simulink model "Car"  (R2022b)
settings: Solver=VariableStepAuto  StartTime=0.0  StopTime=10.0  RelTol=1e-3
libraries: slpidlib x1
settings Model: Creator=Shayan  LastModifiedBy=Shayan
settings DebuggingCC: UnderSpecifiedDimensionMsg=error

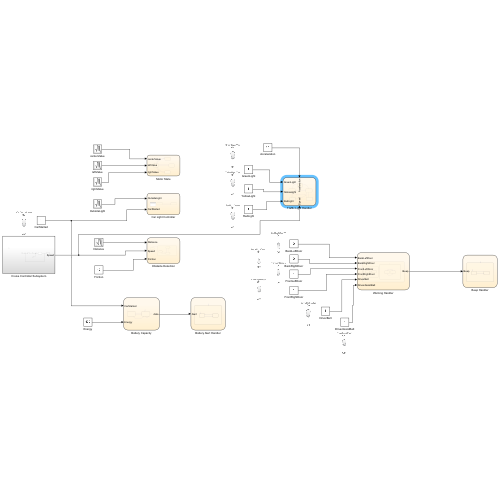
[thumbnail: Simulink's stored preview of the top-level diagram]
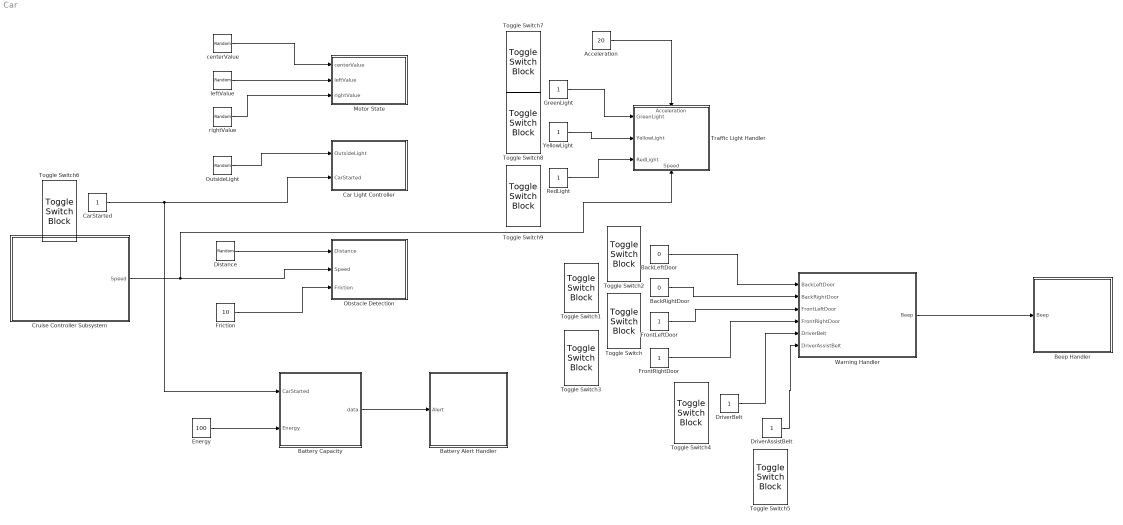
== system Car ==
  Acceleration : Constant  Value=20
  BackLeftDoor : Constant  Value=0
  BackRightDoor : Constant  Value=0
  Battery Alert Handler : Stateflow chart  TreatAsAtomicUnit=on
  Battery Capacity : Stateflow chart  TreatAsAtomicUnit=on
  Beep Handler : Stateflow chart  TreatAsAtomicUnit=on
  Car Light Controller : Stateflow chart  TreatAsAtomicUnit=on
  CarStarted : Constant
  Cruise Controller Subsystem : Subsystem
  Distance : RandomNumber  Mean=1000  Variance=1000  SampleTime=0.1
  DriverAssistBelt : Constant
  DriverBelt : Constant
  Energy : Constant  Value=100
  Friction : Constant  Value=10
  FrontLeftDoor : Constant
  FrontRightDoor : Constant
  GreenLight : Constant
  Motor State : Stateflow chart  TreatAsAtomicUnit=on
  Obstacle Detection : Stateflow chart  TreatAsAtomicUnit=on
  OutsideLight : RandomNumber  Mean=42  Variance=42  SampleTime=0.1
  RedLight : Constant
  Toggle Switch{,1..9} (10 alike) : ToggleSwitchBlock
      settings: Values={{'Off', 'On'}, [0 1]}
  Traffic Light Handler : Stateflow chart  TreatAsAtomicUnit=on
      settings: PortSchema="{\"entries\":[{\"content\":{\"sides\":[{\"content\":{\"connectorIds\":[\"In3\",\"In4\",\"In5\"]},\"type\":\"ConnectorPlacement.EquallySpacedRectSide\",\"uuid\":\"e4f34f1e-9e28-49a6-bd7a-caceeee8cccd\"},{\"content\":{\"connectorIds\":[],\"side\":\"RIGHT\"},\"type\":\"ConnectorPlacement.EquallySpacedRectSide\",\"uuid\":\"aeae50c0-f1a7-40b1-b3c2-19e804339cd4\"},{\"content\":{\"connectorIds\":[\"In2\"],\"side\":\"TOP\"},\"type\":\"ConnectorPlacement.EquallySpacedRectSide\",\"uuid\":\"3a2223b1-1d71-4724-b5b0-9d54e358279c\"},{\"content\":{\"connectorIds\":[\"In1\"],\"side\":\"BOTTOM\"},\"type\":\"ConnectorPlacement.EquallySpacedRectSide\",\"uuid\":\"a90961ba-64bb-42d5-9d38-2be5e1d23df0\"}]},\"type\":\"ConnectorPlacement.EquallySpacedConnector\",\"uuid\":\"7488e4b5-f75e-467c-b059-ab59c8ff95b9\"}],\"packageUris\":[\"http://schema.mathworks.com/mf0/Connector/R2020b\"],\"version\":\"1.0\"}"
  Warning Handler : Stateflow chart  TreatAsAtomicUnit=on
  YellowLight : Constant
  centerValue : RandomNumber  SampleTime=0.1
  leftValue : RandomNumber  SampleTime=0.1
  rightValue : RandomNumber  SampleTime=0.1
  wires:
  OutsideLight/1 -> Car Light Controller/1(OutsideLight)
  Distance/1 -> Obstacle Detection/1(Distance)
  centerValue/1 -> Motor State/1(centerValue)
  leftValue/1 -> Motor State/2(leftValue)
  rightValue/1 -> Motor State/3(rightValue)
  BackLeftDoor/1 -> Warning Handler/1(BackLeftDoor)
  BackRightDoor/1 -> Warning Handler/2(BackRightDoor)
  FrontLeftDoor/1 -> Warning Handler/3(FrontLeftDoor)
  FrontRightDoor/1 -> Warning Handler/4(FrontRightDoor)
  DriverBelt/1 -> Warning Handler/5(DriverBelt)
  DriverAssistBelt/1 -> Warning Handler/6(DriverAssistBelt)
  Warning Handler/1(Beep) -> Beep Handler/1(Beep)
  GreenLight/1 -> Traffic Light Handler/3(GreenLight)
  YellowLight/1 -> Traffic Light Handler/4(YellowLight)
  RedLight/1 -> Traffic Light Handler/5(RedLight)
  Friction/1 -> Obstacle Detection/3(Friction)
  Acceleration/1 -> Traffic Light Handler/2(Acceleration)
  Cruise Controller Subsystem/1(Speed) -> Traffic Light Handler/1(Speed), Obstacle Detection/2(Speed)
  Battery Capacity/1(data) -> Battery Alert Handler/1(Alert)
  Energy/1 -> Battery Capacity/2(Energy)
  CarStarted/1 -> Car Light Controller/2(CarStarted), Battery Capacity/1(CarStarted)

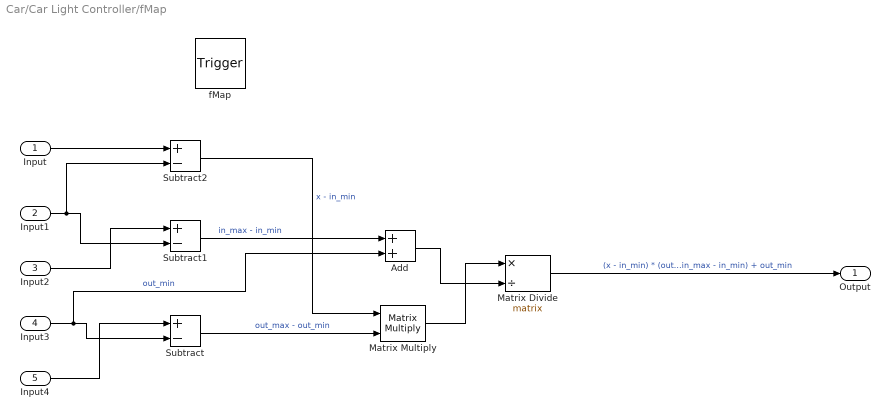
== system Car/Car Light Controller/fMap ==
  Input : Inport
  Input1 : Inport  Port=2
  Input2 : Inport  Port=3
  Input3 : Inport  Port=4
  Input4 : Inport  Port=5
  fMap : TriggerPort  TriggerType=function-call  VariantControl=(inherit)
      settings: CopyFcn=Stateflow.SLINSF.SimulinkMan.removeBlockPreDeleteFcn  PreDeleteFcn=Stateflow.SLINSF.SimulinkMan.unsafePredeleteFcn
  Add : Sum
  Matrix Divide : Product  Inputs=*/  Multiplication=Matrix(*)
  Matrix Multiply : Product  Multiplication=Matrix(*)
  Subtract : Sum  Inputs=+-
  Subtract1 : Sum  Inputs=+-
  Subtract2 : Sum  Inputs=+-
  Output : Outport
  wires:
  Input4/1 -> Subtract/1
  Input3/1 -> Add/2, Subtract/2  "out_min"
  Input2/1 -> Subtract1/1
  Input1/1 -> Subtract2/2, Subtract1/2
  Input/1 -> Subtract2/1
  Subtract2/1 -> Matrix Multiply/1  "x - in_min"
  Subtract/1 -> Matrix Multiply/2  "out_max - out_min"
  Subtract1/1 -> Add/1  "in_max - in_min"
  Matrix Multiply/1 -> Matrix Divide/1
  Add/1 -> Matrix Divide/2
  Matrix Divide/1 -> Output/1  "(x - in_min) * (out_max - out_min) / (in_max - in_min) + out_min"

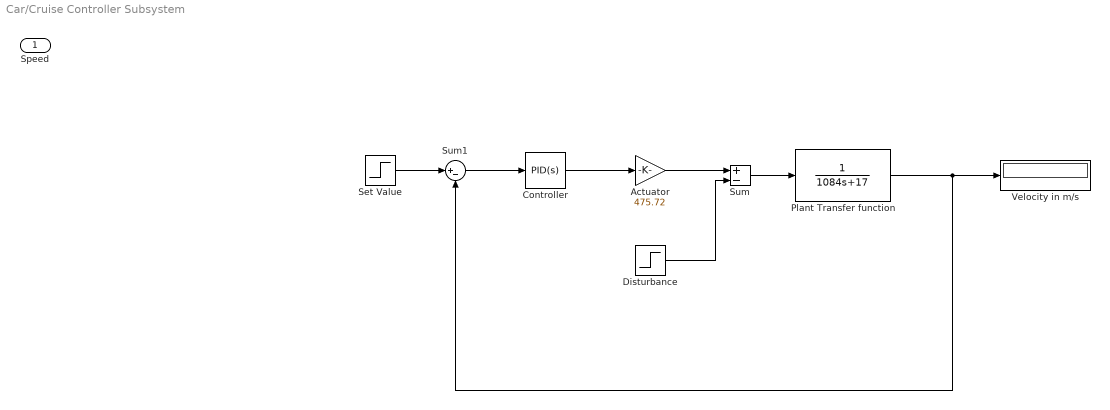
== system Car/Cruise Controller Subsystem ==
  Actuator : Gain  Gain=475.72
  Controller : slpidlib/PID Controller  Controller=PID  Form=Parallel  TimeDomain=Continuous-time  UseExternalTs=off  SampleTime=-1  IntegratorMethod=Forward Euler  FilterMethod=Forward Euler  ControllerParametersSource=internal  P=.27  I=.012  UseKiTs=off  D=.21  N=.21  UseFilter=on  TunerSelectOption=Transfer Function Based (PID Tuner App)  InitialConditionSource=internal  InitialConditionForIntegrator=0  InitialConditionForFilter=0  DifferentiatorICPrevScaledInput=0  ExternalReset=none  TrackingMode=off  Kt=1  LimitOutput=off  SatLimitsSource=internal  UpperSaturationLimit=inf  LowerSaturationLimit=-inf  LinearizeAsGain=on  AntiWindupMode=none  Kb=1  LimitIntegrator=off  UpperIntegratorSaturationLimit=inf  LowerIntegratorSaturationLimit=-inf  POutMin=[]  POutMax=[]  IOutMin=[]  IOutMax=[]  DOutMin=[]  DOutMax=[]  NOutMin=[]  NOutMax=[]  SumOutMin=[]  SumOutMax=[]  SaturationOutMin=[]  SaturationOutMax=[]  PParamMin=[]  PParamMax=[]  IParamMin=[]  IParamMax=[]  DParamMin=[]  DParamMax=[]  NParamMin=[]  NParamMax=[]  KbParamMin=[]  KbParamMax=[]  KtParamMin=[]  KtParamMax=[]  KbOutMin=[]  KbOutMax=[]  KtOutMin=[]  KtOutMax=[]  IntegratorOutMin=[]  IntegratorOutMax=[]  FilterOutMin=[]  FilterOutMax=[]  SumI1OutMin=[]  SumI1OutMax=[]  SumI2OutMin=[]  SumI2OutMax=[]  SumI3OutMin=[]  SumI3OutMax=[]  SumI4OutMin=[]  SumI4OutMax=[]  SumDOutMin=[]  SumDOutMax=[]  DifferentiatorOutMin=[]  DifferentiatorOutMax=[]  FilterDiffOutCoefMin=[]  FilterDiffOutCoefMax=[]  ReciprocalOutMin=[]  ReciprocalOutMax=[]  SumDenOutMin=[]  SumDenOutMax=[]  SumNumOutMin=[]  SumNumOutMax=[]  DivideOutMin=[]  DivideOutMax=[]  UdiffTsProdOutMin=[]  UdiffTsProdOutMax=[]  NTsProdOutMin=[]  NTsProdOutMax=[]  UintegralTsProdOutMin=[]  UintegralTsProdOutMax=[]  UngainTsProdOutMin=[]  UngainTsProdOutMax=[]  ClampingZeroOutDataTypeStr=Inherit: Inherit via back propagation  ClampingZeroOutMin=[]  ClampingZeroOutMax=[]  FilterDenConstantOutDataTypeStr=Inherit: Inherit via back propagation  FilterDenConstantOutMin=[]  FilterDenConstantOutMax=[]  PCopyOutDataTypeStr=Inherit: Inherit via back propagation  PCopyOutMin=[]  PCopyOutMax=[]  NCopyOutDataTypeStr=Inherit: Inherit via back propagation  NCopyOutMin=[]  NCopyOutMax=[]  IntegratorContinuousStateAttributes=''  IntegratorStateMustResolveToSignalObject=off  IntegratorRTWStateStorageClass=Auto  FilterContinuousStateAttributes=''  FilterStateMustResolveToSignalObject=off  FilterRTWStateStorageClass=Auto  ParallelPVariant=InternalParameters  IdealPVariant=Disabled  IVariant=InternalParameters  DVariant=InternalParameters  IntegratorVariant=Continuous  SatVariant=Disabled  AWVariant=Passthrough  PCopyVariant=Disabled  TRVariant=Disabled  FdbkBlocksVariant=Forward  IdealPFdbkVariant=Disabled  SatFdbkVariant=Disabled  DerivativeFilterVariant=ContFilter  NVariant=InternalParameters  NCopyVariant=Disabled  FilterICVariant=InternalICsFilter  IntegratorICVariant=InternalICs  ExternalResetVariant=Disabled  TRSumVariant=Passthrough  SumFdbkVariant=Disabled  SumVariant=Sum_PID  TsampFilterVariant=InternalTs  TsampNgainVariant=Passthrough  TsampIntegralVariant=Passthrough  ExternalSaturationOutDataTypeStr=Inherit: Same as second input
  Disturbance : Step  Time=350  After=475.72*9.81*sin(pi/45)  SampleTime=0
  Plant Transfer function : TransferFcn  Denominator=[1084 17]
  Set Value : Step  After=27.78  SampleTime=0
  Sum : Sum  Inputs=+-
  Sum1 : Sum  Inputs=|+-
  Velocity in m/s : Display
  Speed : Outport
  wires:
  Controller/1 -> Actuator/1
  Sum1/1 -> Controller/1
  Sum/1 -> Plant Transfer function/1
  Disturbance/1 -> Sum/2
  Plant Transfer function/1 -> Velocity in m/s/1, Sum1/2
  Set Value/1 -> Sum1/1
  Actuator/1 -> Sum/1

== stateflow chart Car/Car Light Controller ==
  state Output = fMap(Input,Input1,Input2,Input3,Input4) [function]
  state LIGHT_OFF
    during:
    CarLightValue = fMap(OutsideLight, 6, 679, 0, 255);
  state LIGHT_ON
    during:
    CarLightValue = fMap(OutsideLight, 6, 679, 0, 255);
  (default) -> LIGHT_OFF
  LIGHT_OFF -> LIGHT_ON : [CarLightValue >= 127 && CarStarted == 1]{LightOn = 1}
  LIGHT_ON -> LIGHT_OFF : [CarLightValue <= 127 || CarStarted == 0]{LightOn = 0}
  data: Input function_input; Input1 function_input; Input2 function_input; Input3 function_input; Input4 function_input; Output function_output; OutsideLight input; CarStarted input

== stateflow chart Car/Battery Capacity ==
  state NotConsuming
    Alert = 0
  state Consuming
  Consuming -> Consuming [order 3] : after(1, minute){Energy = Energy - 0.1}
  (default) -> NotConsuming
  Consuming -> Consuming [order 5] : [Energy >= 20]{Alert = 0}
  NotConsuming -> Consuming : [CarStarted == 1]
  Consuming -> NotConsuming [order 1] : [CarStarted == 0]
  Consuming -> NotConsuming [order 2] : [Energy == 0]{CarStarted = 0}
  Consuming -> Consuming [order 4] : [Energy < 20]{Alert = 1}
  data: CarStarted input; data output; Energy input

== stateflow chart Car/Battery Alert Handler ==
  state AlertLED
    state AlertOff
      during:
      turnOffLED();
    state AlertOn
      during:
      turnOnLED();
    (default) -> AlertOff
    AlertOn -> AlertOff : [Alert == 0]
    AlertOff -> AlertOn : [Alert == 1]
  (default) -> AlertLED
  data: Alert input

== stateflow chart Car/Traffic Light Handler ==
  state Stopped
  state Moving
  state FullyStop
    during:
    Speed = Speed - Friction * 1;
  state StartMoving
    during:
    Speed = Speed + Acceleration
  state SlowDown
    during:
    Speed = Speed - Friction * 0.5;
  (default) -> Stopped
  Stopped -> Moving : [Speed > 0]
  FullyStop -> Stopped [order 2] : [Speed == 0]
  Moving -> FullyStop [order 2] : [redLight == 1]
  StartMoving -> Moving : [greenLight == 1 || Speed > 100]
  Moving -> StartMoving [order 3] : [yellowLight == 1 && Speed == 0]
  Moving -> SlowDown [order 1] : [yellowLight == 1 && Speed > 0]
  FullyStop -> StartMoving [order 1] : [yellowLight == 1]
  SlowDown -> FullyStop : [redLight == 1]
  data: Speed input; Acceleration input; GreenLight input; YellowLight input; RedLight input

== stateflow chart Car/Warning Handler ==
  state WarningSystem
    state DoorChecker
      state DoorOpen
      state DoorsClosed
      DoorOpen -> DoorsClosed : [BackLeftDoor == 1 && BackRightDoor == 1 && FrontLeftDoor == 1 && FrontRightDoor == 1]{Beep = 0}
      (default) -> DoorsClosed
      DoorsClosed -> DoorOpen : [BackLeftDoor == 0 || BackRightDoor == 0 || FrontLeftDoor == 0 && FrontRightDoor == 0]{Beep = 1}
    state SeatBeltCecker
      state BeltUntighted
      state BeltTighted
      (default) -> BeltTighted
      BeltTighted -> BeltUntighted : [DriverBelt == 0 || DriverAssistBelt == 0]{Beep = 1}
      BeltUntighted -> BeltTighted : [DriverBelt == 1 && DriverAssistBelt == 1]{Beep = 1}
    (default) -> DoorChecker [order 2]
    (default) -> SeatBeltCecker [order 1]
  (default) -> WarningSystem
  data: BackLeftDoor input; BackRightDoor input; FrontLeftDoor input; FrontRightDoor input; DriverBelt input; DriverAssistBelt input; Beep output

== stateflow chart Car/Beep Handler ==
  state BeepPlayer
    state BeepOff
      turnOffBeep();
    state BeepOn
      during:
      playBeep();
    (default) -> BeepOff
    BeepOn -> BeepOff : [Beep == 0]
    BeepOff -> BeepOn : [Beep == 1]
  (default) -> BeepPlayer
  data: Beep input

== stateflow chart Car/Motor State ==
  state turnLeft
    entry:
    IN1 = 0 ;
    IN2 = 1;
    IN3 = 1;
    IN4 = 0;
  state stopMotor
    entry:
    IN1 = 0;
    IN2 = 0;
    IN3 = 0;
    IN4 = 0;
  state turnRight
    entry:
    IN1 = 1;
    IN2 = 0;
    IN3 = 0;
    IN4 = 1;
  state goForward
    entry:
    IN1 = 1;
    IN2 = 0;
    IN3 = 1;
    IN4 = 0;
  stopMotor -> turnLeft [order 1] : after(20,miliseconds)[leftValue > 500]
  turnLeft -> stopMotor : after(20,miliseconds)[leftValue < 500]
  (default) -> stopMotor
  turnRight -> stopMotor : after(20,miliseconds)[rightValue < 500]
  stopMotor -> turnRight [order 2] : after(20,miliseconds)[rightValue > 500]
  goForward -> stopMotor : after(20,miliseconds)[centerValue < 500]
  stopMotor -> goForward [order 3] : after(20,miliseconds)[centerValue > 500]
  data: centerValue input; leftValue input; rightValue input

== stateflow chart Car/Obstacle Detection ==
  state Moving
    state KILLING
    state SAFE
    state DANGEROUS
    KILLING -> KILLING [order 2] : [Speed > 0]{Speed = Speed - Friction}
    DANGEROUS -> KILLING [order 1] : [Speed >= Distance / 2]{Brake = 1}
    KILLING -> DANGEROUS [order 1] : [Speed < Distance / 2]{Brake = 0.5}
    (default) -> SAFE
    DANGEROUS -> SAFE [order 3] : [Speed < Distance / 10]{Brake = 0}
    SAFE -> DANGEROUS : [Speed >= Distance / 10]{Brake = 0.5}
    DANGEROUS -> DANGEROUS [order 2] : [Speed < Distance / 2]{Speed = Speed - (Brake * Friction)}
  state Stopped
  Stopped -> Moving : [Speed ~= 0]
  (default) -> Stopped
  Moving -> Stopped : [Speed == 0]
  data: Distance input; Speed input; Friction input
